simulink model "Simulink_PID_2021"  (R2021b)
settings: Solver=VariableStepAuto  StartTime=0.0  StopTime=10.0  RelTol=1e-3
undefined symbols (not defined in the file or in its folder): i0, Ke, Kg, Kt, L, R
libraries: slpidlib x2
settings Model: Creator=willf  LastModifiedBy=willf
settings DebuggingCC: UnconnectedInputMsg=none  UnconnectedOutputMsg=none  UnconnectedLineMsg=none
settings ModelReferenceCC: EnableRefExpFcnMdlSchedulingChecks=off
settings RTWCC: DLArmComputeVersion=20.02.1

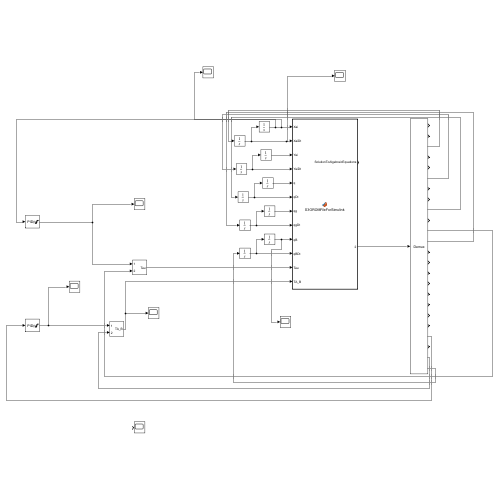
[thumbnail: Simulink's stored preview of the top-level diagram]
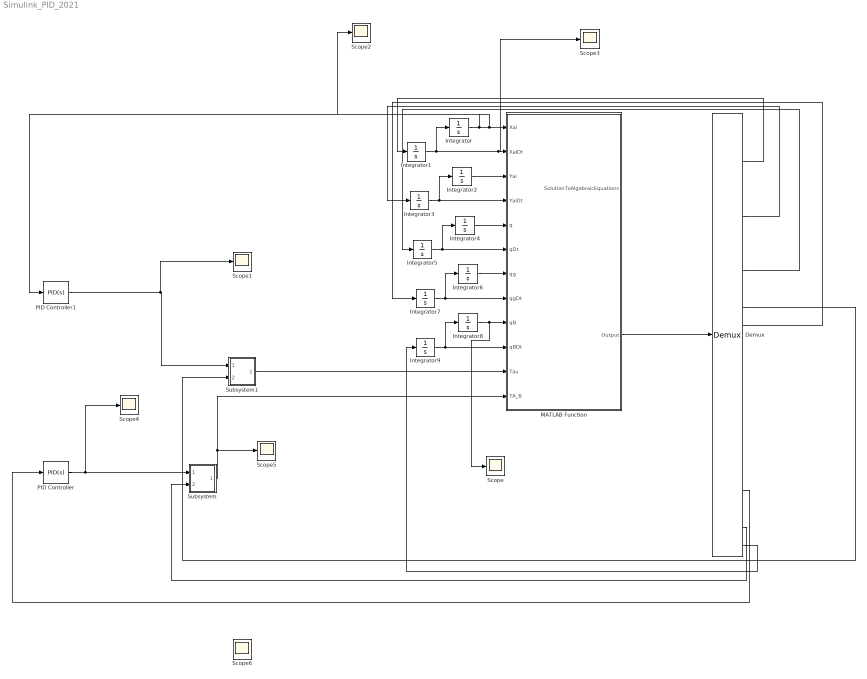
== system Simulink_PID_2021 ==
  Demux : Demux  Outputs=24
      settings: DisplayOption=none
  Integrator{,1..9} (10 alike) : Integrator
  MATLAB Function : MATLAB Function  TreatAsAtomicUnit=on
  PID Controller : slpidlib/PID Controller  Controller=PID  Form=Parallel  TimeDomain=Continuous-time  UseExternalTs=off  SampleTime=-1  IntegratorMethod=Forward Euler  FilterMethod=Forward Euler  ControllerParametersSource=internal  P=80  I=20000  D=10  N=100  UseFilter=on  TunerSelectOption=Transfer Function Based (PID Tuner App)  InitialConditionSource=internal  InitialConditionForIntegrator=0  InitialConditionForFilter=0  DifferentiatorICPrevScaledInput=0  ExternalReset=none  TrackingMode=off  Kt=1  LimitOutput=on  SatLimitsSource=internal  UpperSaturationLimit=12  LowerSaturationLimit=-12  LinearizeAsGain=on  AntiWindupMode=none  Kb=1  POutMin=[]  POutMax=[]  IOutMin=[]  IOutMax=[]  DOutMin=[]  DOutMax=[]  NOutMin=[]  NOutMax=[]  SumOutMin=[]  SumOutMax=[]  SaturationOutMin=[]  SaturationOutMax=[]  PParamMin=[]  PParamMax=[]  IParamMin=[]  IParamMax=[]  DParamMin=[]  DParamMax=[]  NParamMin=[]  NParamMax=[]  KbParamMin=[]  KbParamMax=[]  KtParamMin=[]  KtParamMax=[]  KbOutMin=[]  KbOutMax=[]  KtOutMin=[]  KtOutMax=[]  IntegratorOutMin=[]  IntegratorOutMax=[]  FilterOutMin=[]  FilterOutMax=[]  SumI1OutMin=[]  SumI1OutMax=[]  SumI2OutMin=[]  SumI2OutMax=[]  SumI3OutMin=[]  SumI3OutMax=[]  SumI4OutMin=[]  SumI4OutMax=[]  SumDOutMin=[]  SumDOutMax=[]  DifferentiatorOutMin=[]  DifferentiatorOutMax=[]  FilterDiffOutCoefMin=[]  FilterDiffOutCoefMax=[]  ReciprocalOutMin=[]  ReciprocalOutMax=[]  SumDenOutMin=[]  SumDenOutMax=[]  SumNumOutMin=[]  SumNumOutMax=[]  DivideOutMin=[]  DivideOutMax=[]  UdiffTsProdOutMin=[]  UdiffTsProdOutMax=[]  NTsProdOutMin=[]  NTsProdOutMax=[]  UintegralTsProdOutMin=[]  UintegralTsProdOutMax=[]  UngainTsProdOutMin=[]  UngainTsProdOutMax=[]  IntegratorContinuousStateAttributes=''  IntegratorStateMustResolveToSignalObject=off  IntegratorRTWStateStorageClass=Auto  FilterContinuousStateAttributes=''  FilterStateMustResolveToSignalObject=off  FilterRTWStateStorageClass=Auto  ParallelPVariant=InternalParameters  IdealPVariant=Disabled  IVariant=InternalParameters  DVariant=InternalParameters  IntegratorVariant=Continuous  SatVariant=Enabled  AWVariant=Passthrough  PCopyVariant=Disabled  TRVariant=Disabled  FdbkBlocksVariant=Forward  IdealPFdbkVariant=Disabled  SatFdbkVariant=Disabled  DerivativeFilterVariant=ContFilter  NVariant=InternalParameters  NCopyVariant=Disabled  FilterICVariant=InternalICsFilter  IntegratorICVariant=InternalICs  ExternalResetVariant=Disabled  TRSumVariant=Passthrough  SumFdbkVariant=Disabled  SumVariant=Sum_PID  TsampFilterVariant=InternalTs  TsampNgainVariant=Passthrough  TsampIntegralVariant=Disabled_SignalSpec  ExternalSaturationOutDataTypeStr=Inherit: Same as second input
  PID Controller1 : slpidlib/PID Controller  Controller=PID  Form=Parallel  TimeDomain=Continuous-time  UseExternalTs=off  SampleTime=-1  IntegratorMethod=Forward Euler  FilterMethod=Forward Euler  ControllerParametersSource=internal  P=1  I=1  D=0.5  N=100  UseFilter=on  TunerSelectOption=Transfer Function Based (PID Tuner App)  InitialConditionSource=internal  InitialConditionForIntegrator=0  InitialConditionForFilter=0  DifferentiatorICPrevScaledInput=0  ExternalReset=none  TrackingMode=off  Kt=1  LimitOutput=on  SatLimitsSource=internal  UpperSaturationLimit=12  LowerSaturationLimit=-12  LinearizeAsGain=on  AntiWindupMode=none  Kb=1  POutMin=[]  POutMax=[]  IOutMin=[]  IOutMax=[]  DOutMin=[]  DOutMax=[]  NOutMin=[]  NOutMax=[]  SumOutMin=[]  SumOutMax=[]  SaturationOutMin=[]  SaturationOutMax=[]  PParamMin=[]  PParamMax=[]  IParamMin=[]  IParamMax=[]  DParamMin=[]  DParamMax=[]  NParamMin=[]  NParamMax=[]  KbParamMin=[]  KbParamMax=[]  KtParamMin=[]  KtParamMax=[]  KbOutMin=[]  KbOutMax=[]  KtOutMin=[]  KtOutMax=[]  IntegratorOutMin=[]  IntegratorOutMax=[]  FilterOutMin=[]  FilterOutMax=[]  SumI1OutMin=[]  SumI1OutMax=[]  SumI2OutMin=[]  SumI2OutMax=[]  SumI3OutMin=[]  SumI3OutMax=[]  SumI4OutMin=[]  SumI4OutMax=[]  SumDOutMin=[]  SumDOutMax=[]  DifferentiatorOutMin=[]  DifferentiatorOutMax=[]  FilterDiffOutCoefMin=[]  FilterDiffOutCoefMax=[]  ReciprocalOutMin=[]  ReciprocalOutMax=[]  SumDenOutMin=[]  SumDenOutMax=[]  SumNumOutMin=[]  SumNumOutMax=[]  DivideOutMin=[]  DivideOutMax=[]  UdiffTsProdOutMin=[]  UdiffTsProdOutMax=[]  NTsProdOutMin=[]  NTsProdOutMax=[]  UintegralTsProdOutMin=[]  UintegralTsProdOutMax=[]  UngainTsProdOutMin=[]  UngainTsProdOutMax=[]  IntegratorContinuousStateAttributes=''  IntegratorStateMustResolveToSignalObject=off  IntegratorRTWStateStorageClass=Auto  FilterContinuousStateAttributes=''  FilterStateMustResolveToSignalObject=off  FilterRTWStateStorageClass=Auto  ParallelPVariant=InternalParameters  IdealPVariant=Disabled  IVariant=InternalParameters  DVariant=InternalParameters  IntegratorVariant=Continuous  SatVariant=Enabled  AWVariant=Passthrough  PCopyVariant=Disabled  TRVariant=Disabled  FdbkBlocksVariant=Forward  IdealPFdbkVariant=Disabled  SatFdbkVariant=Disabled  DerivativeFilterVariant=ContFilter  NVariant=InternalParameters  NCopyVariant=Disabled  FilterICVariant=InternalICsFilter  IntegratorICVariant=InternalICs  ExternalResetVariant=Disabled  TRSumVariant=Passthrough  SumFdbkVariant=Disabled  SumVariant=Sum_PID  TsampFilterVariant=InternalTs  TsampNgainVariant=Passthrough  TsampIntegralVariant=Disabled_SignalSpec  ExternalSaturationOutDataTypeStr=Inherit: Same as second input
  Scope{,1..6} (7 alike) : Scope
  Subsystem : Subsystem
  Subsystem1 : Subsystem
  wires:
  MATLAB Function/2(Output) -> Demux/1
  Integrator/1 -> PID Controller1/1, Scope2/1, MATLAB Function/1(Xai)
  Integrator1/1 -> Scope3/1, MATLAB Function/2(XaiDt), Integrator/1
  Demux/3 -> Integrator1/1
  Integrator3/1 -> MATLAB Function/4(YaiDt), Integrator2/1
  Integrator2/1 -> MATLAB Function/3(Yai)
  Demux/6 -> Integrator3/1
  Integrator5/1 -> MATLAB Function/6(qDt), Integrator4/1
  Integrator4/1 -> MATLAB Function/5(q)
  Demux/9 -> Integrator5/1
  Integrator6/1 -> MATLAB Function/7(qg)
  Demux/12 -> Integrator7/1
  Integrator9/1 -> MATLAB Function/10(qBDt), Integrator8/1
  Demux/24 -> Integrator9/1
  PID Controller/1 -> Scope4/1, Subsystem/1(In1)
  Subsystem/1(TA_B) -> MATLAB Function/12(TA_B), Scope5/1
  Integrator7/1 -> MATLAB Function/8(qgDt), Integrator6/1
  PID Controller1/1 -> Scope1/1, Subsystem1/1(In1)
  Demux/11 -> Subsystem1/2(In2)
  Demux/21 -> PID Controller/1
  Demux/23 -> Subsystem/2(In2)
  Subsystem1/1(Tau) -> MATLAB Function/11(Tau)
  Integrator8/1 -> Scope/1, MATLAB Function/9(qB)

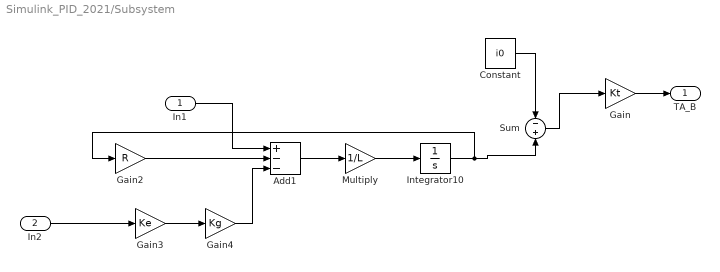
== system Simulink_PID_2021/Subsystem ==
  In1 : Inport
  In2 : Inport  Port=2
  Add1 : Sum  Inputs=+--
  Constant : Constant  Value=i0
  Gain : Gain  Gain=Kt
  Gain2 : Gain  Gain=R
  Gain3 : Gain  Gain=Ke
  Gain4 : Gain  Gain=Kg
  Integrator10 : Integrator
  Multiply : Gain  Gain=1/L
  Sum : Sum  Inputs=-+
  TA_B : Outport
  wires:
  Integrator10/1 -> Sum/2, Gain2/1
  Gain2/1 -> Add1/2
  Multiply/1 -> Integrator10/1
  Gain4/1 -> Add1/3
  Gain/1 -> TA_B/1
  In1/1 -> Add1/1
  Add1/1 -> Multiply/1
  In2/1 -> Gain3/1
  Gain3/1 -> Gain4/1
  Sum/1 -> Gain/1
  Constant/1 -> Sum/1

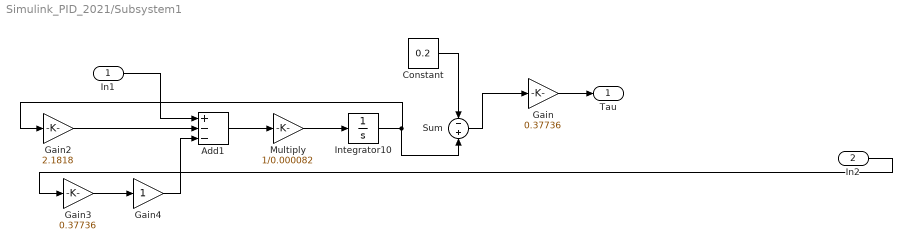
== system Simulink_PID_2021/Subsystem1 ==
  In1 : Inport
  In2 : Inport  Port=2
  Add1 : Sum  Inputs=+--
  Constant : Constant  Value=0.2
  Gain : Gain  Gain=0.37736
  Gain2 : Gain  Gain=2.1818
  Gain3 : Gain  Gain=0.37736
  Gain4 : Gain
  Integrator10 : Integrator
  Multiply : Gain  Gain=1/0.000082
  Sum : Sum  Inputs=-+
  Tau : Outport
  wires:
  Integrator10/1 -> Sum/2, Gain2/1
  Gain2/1 -> Add1/2
  Multiply/1 -> Integrator10/1
  Gain4/1 -> Add1/3
  Gain/1 -> Tau/1
  In1/1 -> Add1/1
  Add1/1 -> Multiply/1
  In2/1 -> Gain3/1
  Gain3/1 -> Gain4/1
  Sum/1 -> Gain/1
  Constant/1 -> Sum/1

== matlab function Simulink_PID_2021/MATLAB Function ==
  data: Xai input; XaiDt input; Yai input; YaiDt input; q input; qDt input; qg input; qgDt input; qB input; qBDt input; SolutionToAlgebraicEquations output; Tau input; TA_B input; Output output size=24
function [SolutionToAlgebraicEquations,Output] = S3GROMFileForSimulink( Xai, XaiDt, Yai, YaiDt, q, qDt, qg, qgDt, qB, qBDt, Tau, TA_B )
if( nargin ~= 12 ) error( 'S3GROMFileForSimulink expects 12 (not %d) command line arguments.', nargin ),  end
%===========================================================================
% File: S3GROMFileForSimulink.m created Jun 19 2024 by MotionGenesis 6.3.
% Portions copyright (c) 2009-2023 Motion Genesis LLC.  Rights reserved.
% MotionGenesis Student Licensee: William Forcier. (until March 2028).
% Paid-up MotionGenesis Student licensees are granted the right
% to distribute this code for legal student-academic (non-professional) purposes only,
% provided this copyright notice appears in all copies and distributions.
%===========================================================================
% The software is provided "as is", without warranty of any kind, express or    
% implied, including but not limited to the warranties of merchantability or    
% fitness for a particular purpose. In no event shall the authors, contributors,
% or copyright holders be liable for any claim, damages or other liability,     
% whether in an action of contract, tort, or otherwise, arising from, out of, or
% in connection with the software or the use or other dealings in the software. 
%===========================================================================


%-------------------------------+--------------------------+-------------------+-----------------
% Quantity                      | Value                    | Units             | Description
%-------------------------------|--------------------------|-------------------|-----------------
g                               =  9.8;                    % N/kg                Constant
IAzz                            =  403.03;                 % kg*mm^2             Constant
IBzz                            =  403.03;                 % kg*mm^2             Constant
ICzz                            =  7270.62;                % g*mm^2              Constant
IPzz                            =  0.1;                    % kg*m^2              Constant
mA                              =  0.5;                    % kg                  Constant
mB                              =  0.2;                    % kg                  Constant
mC                              =  0.020;                  % kg                  Constant
mD                              =  0.020;                  % kg                  Constant
mP                              =  0.2;                    % kg                  Constant
mPpre                           =  0.1;                    % kg                  Constant
Rc                              =  30;                     % mm                  Constant
Td                              =  0.0;                    % N*m                 Constant
Tp                              =  0.0;                    % N*m                 Constant
X_Ao_To_Acm                     =  76.2;                   % mm                  Constant
X_Ao_To_Ccm                     =  152.40;                 % mm                  Constant
X_Bo_To_Bcm                     =  76.2;                   % mm                  Constant
X_Bo_To_Dcm                     =  152.40;                 % mm                  Constant
X_Po_To_Pcm                     =  100;                    % mm                  Constant
X_Po_To_Ppre                    =  200;                    % mm                  Constant
Y_Ao_To_Acm                     =  0;                      % mm                  Constant
Y_Ao_To_Ccm                     =  0;                      % mm                  Constant
Y_Bo_To_Bcm                     =  0;                      % mm                  Constant
Y_Bo_To_Dcm                     =  0;                      % mm                  Constant
Y_Po_To_Pcm                     =  0;                      % mm                  Constant
Y_Po_To_Ppre                    =  0;                      % mm                  Constant
%-------------------------------+--------------------------+-------------------+-----------------

% Unit conversions.  UnitSystem: kg, meter, second.
IAzz = IAzz * 1.0E-06;                                     %  Converted from kg*mm^2 
IBzz = IBzz * 1.0E-06;                                     %  Converted from kg*mm^2 
ICzz = ICzz * 1.0E-09;                                     %  Converted from g*mm^2 
Rc = Rc * 0.001;                                           %  Converted from mm 
X_Ao_To_Acm = X_Ao_To_Acm * 0.001;                         %  Converted from mm 
X_Ao_To_Ccm = X_Ao_To_Ccm * 0.001;                         %  Converted from mm 
X_Bo_To_Bcm = X_Bo_To_Bcm * 0.001;                         %  Converted from mm 
X_Bo_To_Dcm = X_Bo_To_Dcm * 0.001;                         %  Converted from mm 
X_Po_To_Pcm = X_Po_To_Pcm * 0.001;                         %  Converted from mm 
X_Po_To_Ppre = X_Po_To_Ppre * 0.001;                       %  Converted from mm 
Y_Ao_To_Acm = Y_Ao_To_Acm * 0.001;                         %  Converted from mm 
Y_Ao_To_Ccm = Y_Ao_To_Ccm * 0.001;                         %  Converted from mm 
Y_Bo_To_Bcm = Y_Bo_To_Bcm * 0.001;                         %  Converted from mm 
Y_Bo_To_Dcm = Y_Bo_To_Dcm * 0.001;                         %  Converted from mm 
Y_Po_To_Pcm = Y_Po_To_Pcm * 0.001;                         %  Converted from mm 
Y_Po_To_Ppre = Y_Po_To_Ppre * 0.001;                       %  Converted from mm 

%===========================================================================
COEF = zeros( 16, 16 );
COEF(1,1) = -1;
COEF(1,3) = -1;
COEF(1,5) = 1;
COEF(1,13) = mA;
COEF(1,15) = -0.5*mA*((Y_Ao_To_Acm+Y_Ao_To_Ccm)*cos(0.5*qB)-(X_Ao_To_Acm-X_Ao_To_Ccm)*sin(0.5*qB));
COEF(2,2) = -1;
COEF(2,4) = -1;
COEF(2,6) = 1;
COEF(2,14) = mA;
COEF(2,15) = -0.5*mA*((Y_Ao_To_Acm+Y_Ao_To_Ccm)*sin(0.5*qB)+(X_Ao_To_Acm-X_Ao_To_Ccm)*cos(0.5*qB));
COEF(3,1) = 1;
COEF(3,7) = -1;
COEF(3,13) = mB;
COEF(3,15) = -0.5*mB*(X_Ao_To_Ccm*sin(0.5*qB)+X_Bo_To_Bcm*sin(0.5*qB)+Y_Ao_To_Ccm*cos(0.5*qB)-Y_Bo_To_Bcm*cos(0.5*qB));
COEF(4,2) = 1;
COEF(4,8) = -1;
COEF(4,14) = mB;
COEF(4,15) = 0.5*mB*(X_Ao_To_Ccm*cos(0.5*qB)-X_Bo_To_Bcm*cos(0.5*qB)-Y_Ao_To_Ccm*sin(0.5*qB)-Y_Bo_To_Bcm*sin(0.5*qB));
COEF(5,3) = 1;
COEF(5,9) = -1;
COEF(5,13) = mC;
COEF(6,4) = 1;
COEF(6,10) = -1;
COEF(6,14) = mC;
COEF(7,7) = 1;
COEF(7,13) = mD;
COEF(7,15) = -0.5*mD*(X_Ao_To_Ccm*sin(0.5*qB)+X_Bo_To_Dcm*sin(0.5*qB)+Y_Ao_To_Ccm*cos(0.5*qB)-Y_Bo_To_Dcm*cos(0.5*qB));
COEF(8,8) = 1;
COEF(8,11) = -1;
COEF(8,14) = mD;
COEF(8,15) = 0.5*mD*(X_Ao_To_Ccm*cos(0.5*qB)-X_Bo_To_Dcm*cos(0.5*qB)-Y_Ao_To_Ccm*sin(0.5*qB)-Y_Bo_To_Dcm*sin(0.5*qB));
COEF(9,5) = -1;
COEF(9,12) = (mP*X_Po_To_Pcm+mPpre*X_Po_To_Ppre)*cos(q) - (mP*Y_Po_To_Pcm+mPpre*Y_Po_To_Ppre)*sin(q);
COEF(9,13) = mP + mPpre;
COEF(9,15) = -0.5*(mP+mPpre)*(X_Ao_To_Ccm*sin(0.5*qB)+Y_Ao_To_Ccm*cos(0.5*qB));
COEF(10,6) = -1;
COEF(10,12) = (mP*X_Po_To_Pcm+mPpre*X_Po_To_Ppre)*sin(q) + (mP*Y_Po_To_Pcm+mPpre*Y_Po_To_Ppre)*cos(q);
COEF(10,14) = mP + mPpre;
COEF(10,15) = 0.5*(mP+mPpre)*(X_Ao_To_Ccm*cos(0.5*qB)-Y_Ao_To_Ccm*sin(0.5*qB));
COEF(11,1) = X_Ao_To_Acm*sin(0.5*qB) - Y_Ao_To_Acm*cos(0.5*qB);
COEF(11,2) = -X_Ao_To_Acm*cos(0.5*qB) - Y_Ao_To_Acm*sin(0.5*qB);
COEF(11,3) = (X_Ao_To_Acm-X_Ao_To_Ccm)*sin(0.5*qB) - (Y_Ao_To_Acm+Y_Ao_To_Ccm)*cos(0.5*qB);
COEF(11,4) = -(Y_Ao_To_Acm+Y_Ao_To_Ccm)*sin(0.5*qB) - (X_Ao_To_Acm-X_Ao_To_Ccm)*cos(0.5*qB);
COEF(11,5) = Y_Ao_To_Acm*cos(0.5*qB) - X_Ao_To_Acm*sin(0.5*qB);
COEF(11,6) = X_Ao_To_Acm*cos(0.5*qB) + Y_Ao_To_Acm*sin(0.5*qB);
COEF(11,15) = 0.5*IAzz;
COEF(12,1) = Y_Bo_To_Bcm*cos(0.5*qB) - X_Bo_To_Bcm*sin(0.5*qB);
COEF(12,2) = -X_Bo_To_Bcm*cos(0.5*qB) - Y_Bo_To_Bcm*sin(0.5*qB);
COEF(12,7) = (X_Bo_To_Bcm-X_Bo_To_Dcm)*sin(0.5*qB) - (Y_Bo_To_Bcm-Y_Bo_To_Dcm)*cos(0.5*qB);
COEF(12,8) = (X_Bo_To_Bcm-X_Bo_To_Dcm)*cos(0.5*qB) + (Y_Bo_To_Bcm-Y_Bo_To_Dcm)*sin(0.5*qB);
COEF(12,15) = -0.5*IBzz;
COEF(13,9) = -Rc;
COEF(13,15) = 0.5*ICzz;
COEF(13,16) = -ICzz;
COEF(14,5) = X_Po_To_Pcm*cos(q) - Y_Po_To_Pcm*sin(q);
COEF(14,6) = X_Po_To_Pcm*sin(q) + Y_Po_To_Pcm*cos(q);
COEF(14,12) = IPzz - mPpre*X_Po_To_Ppre*(X_Po_To_Pcm-X_Po_To_Ppre) - mPpre*Y_Po_To_Ppre*(Y_Po_To_Pcm-Y_Po_To_Ppre);
COEF(14,13) = -mPpre*((X_Po_To_Pcm-X_Po_To_Ppre)*cos(q)-(Y_Po_To_Pcm-Y_Po_To_Ppre)*sin(q));
COEF(14,14) = -mPpre*((X_Po_To_Pcm-X_Po_To_Ppre)*sin(q)+(Y_Po_To_Pcm-Y_Po_To_Ppre)*cos(q));
COEF(14,15) = 0.5*mPpre*(Y_Ao_To_Ccm*(X_Po_To_Pcm-X_Po_To_Ppre)*cos(q-0.5*qB)-X_Ao_To_Ccm*(X_Po_To_Pcm-X_Po_To_Ppre)*sin(q-0.5*qB)-  ...
X_Ao_To_Ccm*(Y_Po_To_Pcm-Y_Po_To_Ppre)*cos(q-0.5*qB)-Y_Ao_To_Ccm*(Y_Po_To_Pcm-Y_Po_To_Ppre)*sin(q-0.5*qB));
COEF(15,13) = -1;
COEF(15,16) = Rc;
COEF(16,14) = 1;
RHS = zeros( 1, 16 );
RHS(1) = -0.25*mA*((Y_Ao_To_Acm+Y_Ao_To_Ccm)*sin(0.5*qB)+(X_Ao_To_Acm-X_Ao_To_Ccm)*cos(0.5*qB))*qBDt^2;
RHS(2) = 0.25*mA*((Y_Ao_To_Acm+Y_Ao_To_Ccm)*cos(0.5*qB)*qBDt^2-4*g-(X_Ao_To_Acm-X_Ao_To_Ccm)*sin(0.5*qB)*qBDt^2);
RHS(3) = -0.25*mB*(Y_Ao_To_Ccm*sin(0.5*qB)-X_Ao_To_Ccm*cos(0.5*qB)-X_Bo_To_Bcm*cos(0.5*qB)-Y_Bo_To_Bcm*sin(0.5*qB))*qBDt^2;
RHS(4) = -0.25*mB*(4*g+X_Bo_To_Bcm*sin(0.5*qB)*qBDt^2-X_Ao_To_Ccm*sin(0.5*qB)*qBDt^2-Y_Ao_To_Ccm*cos(0.5*qB)*qBDt^2-Y_Bo_To_Bcm*cos(  ...
0.5*qB)*qBDt^2);
RHS(6) = -g*mC;
RHS(7) = -0.25*mD*(Y_Ao_To_Ccm*sin(0.5*qB)-X_Ao_To_Ccm*cos(0.5*qB)-X_Bo_To_Dcm*cos(0.5*qB)-Y_Bo_To_Dcm*sin(0.5*qB))*qBDt^2;
RHS(8) = -0.25*mD*(4*g+X_Bo_To_Dcm*sin(0.5*qB)*qBDt^2-X_Ao_To_Ccm*sin(0.5*qB)*qBDt^2-Y_Ao_To_Ccm*cos(0.5*qB)*qBDt^2-Y_Bo_To_Dcm*cos(  ...
0.5*qB)*qBDt^2);
RHS(9) = (mP*X_Po_To_Pcm+mPpre*X_Po_To_Ppre)*sin(q)*qDt^2 + (mP*Y_Po_To_Pcm+mPpre*Y_Po_To_Ppre)*cos(q)*qDt^2 + 0.25*X_Ao_To_Ccm*(  ...
mP+mPpre)*cos(0.5*qB)*qBDt^2 - 0.25*Y_Ao_To_Ccm*(mP+mPpre)*sin(0.5*qB)*qBDt^2;
RHS(10) = (mP*Y_Po_To_Pcm+mPpre*Y_Po_To_Ppre)*sin(q)*qDt^2 + 0.25*X_Ao_To_Ccm*(mP+mPpre)*sin(0.5*qB)*qBDt^2 + 0.25*Y_Ao_To_Ccm*(mP+  ...
mPpre)*cos(0.5*qB)*qBDt^2 - g*mP - g*mPpre - (mP*X_Po_To_Pcm+mPpre*X_Po_To_Ppre)*cos(q)*qDt^2;
RHS(11) = Tau - Tp - TA_B;
RHS(12) = TA_B - Td;
RHS(13) = -Tau;
RHS(14) = Tp + g*mPpre*(X_Po_To_Pcm-X_Po_To_Ppre)*sin(q) + g*mPpre*(Y_Po_To_Pcm-Y_Po_To_Ppre)*cos(q) + mPpre*X_Po_To_Ppre*  ...
Y_Po_To_Pcm*qDt^2 + 0.25*mPpre*(X_Ao_To_Ccm*(Y_Po_To_Pcm-Y_Po_To_Ppre)*sin(q-0.5*qB)-X_Ao_To_Ccm*(X_Po_To_Pcm-X_Po_To_Ppre)*cos(q-  ...
0.5*qB)-Y_Ao_To_Ccm*(X_Po_To_Pcm-X_Po_To_Ppre)*sin(q-0.5*qB)-Y_Ao_To_Ccm*(Y_Po_To_Pcm-Y_Po_To_Ppre)*cos(q-0.5*qB))*qBDt^2 -   ...
mPpre*X_Po_To_Pcm*Y_Po_To_Ppre*qDt^2;
SolutionToAlgebraicEquations = COEF \ transpose(RHS);

% Update variables after uncoupling equations
FRx_b_a = SolutionToAlgebraicEquations(1);
FRy_b_a = SolutionToAlgebraicEquations(2);
FRx_c_a = SolutionToAlgebraicEquations(3);
FRy_c_a = SolutionToAlgebraicEquations(4);
FRx_p_a = SolutionToAlgebraicEquations(5);
FRy_p_a = SolutionToAlgebraicEquations(6);
FRx_d_b = SolutionToAlgebraicEquations(7);
FRy_d_b = SolutionToAlgebraicEquations(8);
FRcx = SolutionToAlgebraicEquations(9);
FRcy = SolutionToAlgebraicEquations(10);
FRdy = SolutionToAlgebraicEquations(11);
qDDt = SolutionToAlgebraicEquations(12);
XaiDDt = SolutionToAlgebraicEquations(13);
YaiDDt = SolutionToAlgebraicEquations(14);
qBDDt = SolutionToAlgebraicEquations(15);
qgDDt = SolutionToAlgebraicEquations(16);

y = Yai + X_Ao_To_Ccm*sin(0.5*qB) + Y_Ao_To_Ccm*cos(0.5*qB);
yDt = YaiDt + 0.5*X_Ao_To_Ccm*cos(0.5*qB)*qBDt - 0.5*Y_Ao_To_Ccm*sin(0.5*qB)*qBDt;
yDDt = YaiDDt - 0.25*sin(0.5*qB)*(X_Ao_To_Ccm*qBDt^2+2*Y_Ao_To_Ccm*qBDDt) - 0.25*cos(0.5*qB)*(Y_Ao_To_Ccm*qBDt^2-2*X_Ao_To_Ccm*  ...
qBDDt);
x = Xai + X_Ao_To_Ccm*cos(0.5*qB) - Y_Ao_To_Ccm*sin(0.5*qB);
xDt = XaiDt - 0.5*X_Ao_To_Ccm*sin(0.5*qB)*qBDt - 0.5*Y_Ao_To_Ccm*cos(0.5*qB)*qBDt;
xDDt = XaiDDt + 0.25*sin(0.5*qB)*(Y_Ao_To_Ccm*qBDt^2-2*X_Ao_To_Ccm*qBDDt) - 0.25*cos(0.5*qB)*(X_Ao_To_Ccm*qBDt^2+2*Y_Ao_To_Ccm*  ...
qBDDt);



%===========================================================================
Output = zeros( 1, 24 )';

Output(1) = Xai;
Output(2) = XaiDt;
Output(3) = XaiDDt;
Output(4) = Yai;
Output(5) = YaiDt;
Output(6) = YaiDDt;
Output(7) = q;
Output(8) = qDt;
Output(9) = qDDt;
Output(10) = qg;
Output(11) = qgDt;
Output(12) = qgDDt;
Output(13) = FRcx;
Output(14) = FRcy;
Output(15) = FRdy;
Output(16) = x;
Output(17) = xDt;
Output(18) = xDDt;
Output(19) = y;
Output(20) = yDt;
Output(21) = yDDt;
Output(22) = qB;
Output(23) = qBDt;
Output(24) = qBDDt;

%==============================================
end    % End of function S3GROMFileForSimulink
%==============================================
